simulink model "FSE"  (R2020a)
settings: Solver=ode45  StartTime=0.0  StopTime=2e3  RelTol=1e-3  EnableMultiTasking=on
PreLoadFcn:
  | FSE_PreLoadFcn
undefined symbols (not defined in the file): j
libraries: xbsIndex_r4 x138, dspmlti4 x2, xbsCopyrightNotice_r4 x1
(part 1 of 2)
settings Model: Creator=alexc  LastModifiedBy=viswanad
settings DataIOCC: LimitDataPoints=on  SaveFormat=Array  SignalLoggingSaveFormat=ModelDataLogs  ReturnWorkspaceOutputs=off  SignalLoggingName=sigsOut
settings OptimizationCC: BlockReduction=off  BooleanDataType=off  DefaultParameterBehavior=Inlined  ExpressionDepthLimit=2147483647  InitFltsAndDblsToZero=on  LifeSpan=inf
settings DebuggingCC: SaveWithParameterizedLinksMsg=none  UnderspecifiedInitializationDetection=Classic  MergeDetectMultiDrivingBlocksExec=none  SignalResolutionControl=TryResolveAllWithWarning  MultiTaskDSMMsg=warning  MultiTaskCondExecSysMsg=none  FcnCallInpInsideContextMsg=warning  AllowSymbolicDim=off  StateNameClashWarn=warning  SFUnexpectedBacktrackingDiag=warning  SFNoUnconditionalDefaultTransitionDiag=warning  SFExecutionAtInitializationDiag=none  ArithmeticOperatorsInVariantConditions=warning
settings HardwareCC: ProdBitPerPointer=32  ProdBitPerSizeT=32  ProdBitPerPtrDiffT=32  ProdLargestAtomicFloat=None  ProdIntDivRoundTo=Undefined  ProdEndianess=Unspecified  ProdWordSize=32  ProdHWDeviceType=32-bit Generic  TargetUnknown=on
settings ModelReferenceCC: PropagateSignalLabelsOutOfModel=off
settings SFSimCC: SimUseLocalCustomCode=off  CustomCodeUndefinedFunction=UseInterfaceOnly
settings RTWCC: Description=Generic Real-Time Target  RTWUseLocalCustomCode=off
settings CodeAppCC: StateflowObjectComments=on
settings GRTTargetCC: TargetFcnLib=ansi_tfl_tmw.mat  TargetLangStandard=C89/C90 (ANSI)  CombineOutputUpdateFcns=off  GRTInterface=on
settings ConfigComp: CovMetricSettings=dw  CovHtmlReporting=on  CovSaveCumulativeToWorkspaceVar=on  CovSaveSingleToWorkspaceVar=on  CovExternalEMLEnable=off

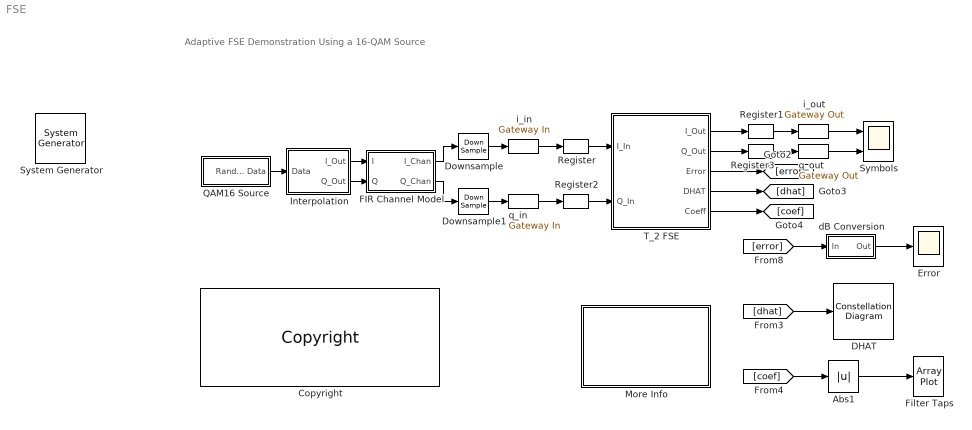
== system FSE ==
  note: Adaptive FSE Demonstration Using a 16-QAM Source
  " System Generator" : xbsIndex_r4/ System Generator  Tag=genX  xilinxfamily=kintex7  part=xc7k325t  speed=-3  package=fbg676  synthesis_tool=Vivado  clock_wrapper=Clock Enables  directory=./netlist  proj_type=Vivado  Synth_file=Vivado Synthesis Defaults  Impl_file=Vivado Implementation Defaults  testbench=off  simulink_period=1  sysclk_period=15  dcm_input_clock_period=10  incr_netlist=off  trim_vbits=Everywhere in SubSystem  dbl_ovrd=According to Block Masks  core_generation=According to Block Masks  run_coregen=off  deprecated_control=off  eval_field=0  block_type=sysgen
  Abs1 : Abs  SaturateOnIntegerOverflow=on
  Copyright : xbsCopyrightNotice_r4/Copyright  copyrighttext="Copyright (c) 2021  by  Xilinx, Inc. All rights reserved.<br><br>This file contains proprietary, confidential information of Xilinx, Inc., is distributed under license from Xilinx, Inc., and may be used, copied and/or disclosed only pursuant to the terms of a valid license agreement with Xilinx, Inc. Xilinx hereby grants you a license to use this file solely for design, simulation, implementation and creation of design files limited to Xilinx devices or technologies. Use with non-Xilinx devices or technologies is expressly prohibited and immediately terminates your license unless covered by a separate agreement.<br><br>Xilinx is providing this design, code, or information \"as-is\" solely for use in developing programs and solutions for Xilinx devices, with no obligation on the part of Xilinx to provide support. By providing this design, code, or information as one possible implementation of this feature, application or standard, Xilinx is making no representation that this implementation is free from any claims of infringement. You are responsible for obtaining any rights you may require for your implementation. Xilinx expressly disclaims any warranty whatsoever with respect to the adequacy of the implementation, including but not limited to any warranties or representations that this implementation is free from claims of infringement, implied warranties of merchantability or fitness for a particular purpose.<br><br>Xilinx products are not intended for use in life support appliances, devices, or systems. Use in such applications is expressly prohibited.<br><br>Any modifications that are made to the Source Code are done at the user's sole risk and will be unsupported.<br><br>This copyright and support notice must be retained as part of this text at all times. (c) Copyright 1995-2021 Xilinx, Inc. All rights reserved."  block_type=copyright
  DHAT : ConstellationDiagram
  Downsample : DownSample  RateOptions=Allow multirate processing
  Downsample1 : DownSample  RateOptions=Allow multirate processing
  Error : Scope
  FIR Channel Model : Subsystem  mask{chan=[1+j*0.1 .2 j*0.2 0 0 0 0 0 0 0]}
      mask prompts: chan "Channel"
  Filter Taps : ArrayPlot
  Interpolation : Subsystem
  More Info : Subsystem
      mask Display: disp('Double click\n for\n more information.')
  QAM16 Source : Subsystem
  Register{,1..3} (4 alike) : xbsIndex_r4/Register  init=0  rst=off  en=off  XmcBlockStatus=1  maskContainerNames=tabcontainer1  block_type=register  block_config=sysgen:Register_config
  Symbols : Scope  NumInputPorts=2
  T_2 FSE : Subsystem  mask{mu=.005}
  dB Conversion : Subsystem
  i_in : xbsIndex_r4/Gateway In  gui_display_data_type=Fixed-point  arith_type=Signed (2's comp)  n_bits=12  bin_pt=10  preci_type=Single  exp_width=8  frac_width=24  rows=1  columns=1  quantization="Round  (unbiased: +/- Inf)"  overflow=Saturate  period=2  UseAsADC=off  ADCChannel='1'  interface=None  automatic_assignment=on  address_offset=hex2dec('00')  intf_name=''  intf_description=''  default_value=0  timing_constraint=None  locs_specified=off  LOCs={}  io_standard={}  inherit_from_input=off  hdl_port=on  XmcBlockStatus=1  maskContainerNames=group4  block_type=gatewayin  block_config=sysgen:gateway_in_config
  i_out : xbsIndex_r4/Gateway Out  inherit_from_input=off  hdl_port=on  rows=1  columns=1  UseAsDAC=off  DACChannel='1'  interface=None  automatic_assignment=on  address_offset=hex2dec('00')  intf_name=''  intf_description=''  timing_constraint="Data Rate;  Set 'FAST' Attribute"  locs_specified=off  LOCs={}  io_standard={}  XmcBlockStatus=1  maskContainerNames=group4  block_type=gatewayout  block_config=sysgen:gateway_out_config
  q_in : xbsIndex_r4/Gateway In  gui_display_data_type=Fixed-point  arith_type=Signed (2's comp)  n_bits=12  bin_pt=10  preci_type=Single  exp_width=8  frac_width=24  rows=1  columns=1  quantization="Round  (unbiased: +/- Inf)"  overflow=Saturate  period=2  UseAsADC=off  ADCChannel='1'  interface=None  automatic_assignment=on  address_offset=hex2dec('00')  intf_name=''  intf_description=''  default_value=0  timing_constraint=None  locs_specified=off  LOCs={}  io_standard={}  inherit_from_input=off  hdl_port=on  XmcBlockStatus=1  maskContainerNames=group4  block_type=gatewayin  block_config=sysgen:gateway_in_config
  q_out : xbsIndex_r4/Gateway Out  inherit_from_input=off  hdl_port=on  rows=1  columns=1  UseAsDAC=off  DACChannel='1'  interface=None  automatic_assignment=on  address_offset=hex2dec('00')  intf_name=''  intf_description=''  timing_constraint="Data Rate;  Set 'FAST' Attribute"  locs_specified=off  LOCs={}  io_standard={}  XmcBlockStatus=1  maskContainerNames=group4  block_type=gatewayout  block_config=sysgen:gateway_out_config
  wires:
  QAM16 Source/1(" Random Data") -> Interpolation/1(Data)
  Interpolation/2(Q_Out) -> FIR Channel Model/2(Q)
  T_2 FSE/3(Error) -> [error]
  Downsample1/1 -> q_in/1
  Downsample/1 -> i_in/1
  Interpolation/1(I_Out) -> FIR Channel Model/1(I)
  T_2 FSE/2(Q_Out) -> Register3/1
  T_2 FSE/1(I_Out) -> Register1/1
  FIR Channel Model/1(I_Chan) -> Downsample/1
  FIR Channel Model/2(Q_Chan) -> Downsample1/1
  T_2 FSE/5(Coeff) -> [coef]
  i_in/1 -> Register/1
  Abs1/1 -> Filter Taps/1
  T_2 FSE/4(DHAT) -> [dhat]
  dB Conversion/1(Out) -> Error/1
  Register2/1 -> T_2 FSE/2(Q_In)
  Register1/1 -> i_out/1
  Register3/1 -> q_out/1
  q_in/1 -> Register2/1
  Register/1 -> T_2 FSE/1(I_In)
  [coef] -> Abs1/1
  [dhat] -> DHAT/1
  [error] -> dB Conversion/1(In)
  i_out/1 -> Symbols/1
  q_out/1 -> Symbols/2

== system FSE/FIR Channel Model ==
  I : Inport
  Q : Inport  Port=2
  Channel : Subsystem
  Channel1 : Subsystem
  Complex to Real-Imag1 : ComplexToRealImag
  Gain : Gain  Gain=j  SaturateOnIntegerOverflow=on  OutDataTypeStr=Inherit: Same as input  ParamDataTypeStr=Inherit: Same as input
  Random Number : RandomNumber  Variance=.01  SampleTime=100000
  Sum : Sum  Inputs=+++  InputSameDT=on  SaturateOnIntegerOverflow=on  OutDataTypeStr=Inherit: Same as first input
  I_Chan : Outport  VectorParamsAs1DForOutWhenUnconnected=off
  Q_Chan : Outport  Port=2  VectorParamsAs1DForOutWhenUnconnected=off
  wires:
  Channel1/1(yn) -> Gain/1
  Channel/1(yn) -> Sum/1
  Q/1 -> Channel1/1(xn)
  I/1 -> Channel/1(xn)
  Random Number/1 -> Sum/2
  Gain/1 -> Sum/3
  Sum/1 -> Complex to Real-Imag1/1
  Complex to Real-Imag1/2 -> Q_Chan/1
  Complex to Real-Imag1/1 -> I_Chan/1

== system FSE/Interpolation ==
  Data : Inport
  Complex to Real-Imag5 : ComplexToRealImag
  FIR Interpolation : dspmlti4/FIR Interpolation  FilterSource=Dialog parameters  PrivateCoeffs=0  h=sinc(-3:.25:3);  L=4  FilterObject=Hm_firinterp  framing=Allow multirate processing  outputBufInitCond=0  roundingMode=Floor  overflowMode=off  firstCoeffDataTypeStr=Inherit: Same word length as input  firstCoeffMin=[]  firstCoeffMax=[]  firstCoeffLastDataTypeStr=Inherit: Same word length as input  outputDataTypeStr=Inherit: Same as accumulator  outputMin=[]  outputMax=[]  outputLastDataTypeStr=Inherit: Same as accumulator
  FIR Interpolation1 : dspmlti4/FIR Interpolation  FilterSource=Dialog parameters  PrivateCoeffs=0  h=sinc(-3:.25:3);  L=4  FilterObject=Hm_firinterp  framing=Allow multirate processing  outputBufInitCond=0  roundingMode=Floor  overflowMode=off  firstCoeffDataTypeStr=Inherit: Same word length as input  firstCoeffMin=[]  firstCoeffMax=[]  firstCoeffLastDataTypeStr=Inherit: Same word length as input  outputDataTypeStr=Inherit: Same as accumulator  outputMin=[]  outputMax=[]  outputLastDataTypeStr=Inherit: Same as accumulator
  I_Out : Outport  VectorParamsAs1DForOutWhenUnconnected=off
  Q_Out : Outport  Port=2  VectorParamsAs1DForOutWhenUnconnected=off
  wires:
  Complex to Real-Imag5/2 -> FIR Interpolation1/1
  Complex to Real-Imag5/1 -> FIR Interpolation/1
  FIR Interpolation/1 -> I_Out/1
  Data/1 -> Complex to Real-Imag5/1
  FIR Interpolation1/1 -> Q_Out/1

== system FSE/More Info ==
  note: This design shows a T/2 adaptive Fractionally Space Equalizer (FSE)
      | operating on a 16-QAM data source with noise and filtering introduced
      | in the channel model.  The two 4-tap FIR filters are based on an
      | SRL16E-based MAC implementation.
      |
      | The DHAT scope provides an X-Y plot of the I and Q filter outputs from
      | within the FSE.  As the simulation progresses, these symbols will
      | converge as the error is reduced.  The magnitude of the filter coefficients
      | is shown in a vector scope as well.  Increasing the simulation duration
      | will allow better visualization of the adaptive FSE effects on the filter output.
      |
      |
      | For additional information on FSE:
      |
      | J.R. Treichler, I. Fijalkow, and C.R. Johnson, Jr.  "Fractionally Spaced
      | Equalizers"  IEEE Signal Processing Magazine, May 1996, pp. 65-81.
      |
      | Chris H. Dick, "Design and implementation of high-performance FPGA
      | signal processing datapaths for software-defined radios" VMEbus
      | Systems, August 2001.
  note: Adaptive FSE Demonstration Using a 16-QAM Source

== system FSE/QAM16 Source ==
  QAM16 - I : Subsystem
  QAM16 -Q : Subsystem
  Real-Imag to Complex : RealImagToComplex
  " Random Data" : Outport  VectorParamsAs1DForOutWhenUnconnected=off
  wires:
  QAM16 - I/1(I) -> Real-Imag to Complex/1
  QAM16 -Q/1(Q) -> Real-Imag to Complex/2
  Real-Imag to Complex/1 -> " Random Data"/1

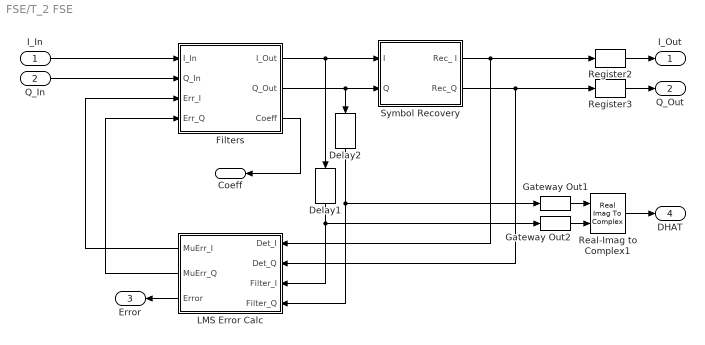
== system FSE/T_2 FSE ==
  I_In : Inport
  Q_In : Inport  Port=2
  Delay1 : xbsIndex_r4/Delay  rst=off  en=off  latency=2  reg_retiming=off  XmcBlockStatus=1  maskContainerNames=group1  block_type=delay  block_config=sysgen:Delay_config
  Delay2 : xbsIndex_r4/Delay  rst=off  en=off  latency=2  reg_retiming=off  XmcBlockStatus=1  maskContainerNames=group1  block_type=delay  block_config=sysgen:Delay_config
  Filters : Subsystem
  Gateway Out1 : xbsIndex_r4/Gateway Out  inherit_from_input=off  hdl_port=off  rows=1  columns=1  UseAsDAC=off  DACChannel='1'  interface=None  automatic_assignment=on  address_offset=hex2dec('00')  intf_name=''  intf_description=''  timing_constraint=None  locs_specified=off  LOCs={}  io_standard={}  XmcBlockStatus=1  maskContainerNames=group4  block_type=gatewayout  block_config=sysgen:gateway_out_config
  Gateway Out2 : xbsIndex_r4/Gateway Out  inherit_from_input=off  hdl_port=off  rows=1  columns=1  UseAsDAC=off  DACChannel='1'  interface=None  automatic_assignment=on  address_offset=hex2dec('00')  intf_name=''  intf_description=''  timing_constraint=None  locs_specified=off  LOCs={}  io_standard={}  XmcBlockStatus=1  maskContainerNames=group4  block_type=gatewayout  block_config=sysgen:gateway_out_config
  LMS Error Calc : Subsystem
  Real-Imag to Complex1 : RealImagToComplex
  Register2 : xbsIndex_r4/Register  init=0  rst=off  en=off  XmcBlockStatus=1  maskContainerNames=tabcontainer1  block_type=register  block_config=sysgen:Register_config
  Register3 : xbsIndex_r4/Register  init=0  rst=off  en=off  XmcBlockStatus=1  maskContainerNames=tabcontainer1  block_type=register  block_config=sysgen:Register_config
  Symbol Recovery : Subsystem
  I_Out : Outport  VectorParamsAs1DForOutWhenUnconnected=off
  Q_Out : Outport  Port=2  VectorParamsAs1DForOutWhenUnconnected=off
  Error : Outport  Port=3  VectorParamsAs1DForOutWhenUnconnected=off
  DHAT : Outport  Port=4  VectorParamsAs1DForOutWhenUnconnected=off
  Coeff : Outport  Port=5  VectorParamsAs1DForOutWhenUnconnected=off
  wires:
  Q_In/1 -> Filters/2(Q_In)
  LMS Error Calc/2(MuErr_Q) -> Filters/4(Err_Q)
  LMS Error Calc/1(MuErr_I) -> Filters/3(Err_I)
  Filters/1(I_Out) -> Delay1/1, Symbol Recovery/1(I)
  Symbol Recovery/2(Rec_Q) -> LMS Error Calc/2(Det_Q), Register3/1
  Symbol Recovery/1(Rec_ I) -> LMS Error Calc/1(Det_I), Register2/1
  Filters/2(Q_Out) -> Symbol Recovery/2(Q), Delay2/1
  I_In/1 -> Filters/1(I_In)
  Delay1/1 -> Gateway Out2/1, LMS Error Calc/3(Filter_I)
  Delay2/1 -> Gateway Out1/1, LMS Error Calc/4(Filter_Q)
  Real-Imag to Complex1/1 -> DHAT/1
  Gateway Out1/1 -> Real-Imag to Complex1/1
  Gateway Out2/1 -> Real-Imag to Complex1/2
  Filters/3(Coeff) -> Coeff/1
  LMS Error Calc/3(Error) -> Error/1
  Register2/1 -> I_Out/1
  Register3/1 -> Q_Out/1

== system FSE/dB Conversion ==
  In : Inport
  Abs : Abs  SaturateOnIntegerOverflow=on
  Constant : Constant  Value=0
  Constant1 : Constant
  Constant2 : Constant
  Gain1 : Gain  Gain=20  SaturateOnIntegerOverflow=on  OutDataTypeStr=Inherit: Same as input  ParamDataTypeStr=Inherit: Same as input
  Multiport Switch : MultiPortSwitch  Inputs=2  SaturateOnIntegerOverflow=on  InputSameDT=on
  Relational Operator : RelationalOperator  Operator===  RndMeth=Nearest  InputSameDT=on
  Sum : Sum  Inputs=|++  InputSameDT=on  SaturateOnIntegerOverflow=on  OutDataTypeStr=Inherit: Same as first input
  log10 : Math  Operator=log10  SignedPower=on  SaturateOnIntegerOverflow=on
  Out : Outport  VectorParamsAs1DForOutWhenUnconnected=off
  wires:
  Multiport Switch/1 -> log10/1
  Constant1/1 -> Multiport Switch/3
  Constant/1 -> Relational Operator/1
  Abs/1 -> Multiport Switch/2, Relational Operator/2
  Constant2/1 -> Sum/2
  Sum/1 -> Multiport Switch/1
  Relational Operator/1 -> Sum/1
  Gain1/1 -> Out/1
  In/1 -> Abs/1
  log10/1 -> Gain1/1

== system FSE/FIR Channel Model/Channel ==
  xn : Inport
  Chan Re : Subsystem
  yn : Outport  VectorParamsAs1DForOutWhenUnconnected=off
  wires:
  xn/1 -> Chan Re/1(Input)
  Chan Re/1(Output) -> yn/1

== system FSE/FIR Channel Model/Channel1 ==
  xn : Inport
  Chan Re : Subsystem
  yn : Outport  VectorParamsAs1DForOutWhenUnconnected=off
  wires:
  xn/1 -> Chan Re/1(Input)
  Chan Re/1(Output) -> yn/1

== system FSE/QAM16 Source/QAM16 - I ==
  Constant : Constant  Value=3
  Gain : Gain  Gain=2  SaturateOnIntegerOverflow=on  OutDataTypeStr=Inherit: Same as input  ParamDataTypeStr=Inherit: Same as input
  Gain1 : Gain  Gain=1/3  SaturateOnIntegerOverflow=on  OutDataTypeStr=Inherit: Same as input  ParamDataTypeStr=Inherit: Same as input
  Random Integer Generator : Subsystem  mask{M=4, seed=1, Ts=4}
      mask prompts: M "M-ary Number"; seed "Initial seed"; Ts "Sample Time"
  Sum : Sum  Inputs=|+-  InputSameDT=on  SaturateOnIntegerOverflow=on  OutDataTypeStr=Inherit: Same as first input
  I : Outport  VectorParamsAs1DForOutWhenUnconnected=off
  wires:
  Random Integer Generator/1(Out1) -> Gain/1
  Gain/1 -> Sum/1
  Constant/1 -> Sum/2
  Sum/1 -> Gain1/1
  Gain1/1 -> I/1

== system FSE/QAM16 Source/QAM16 -Q ==
  Constant : Constant  Value=3
  Gain : Gain  Gain=2  SaturateOnIntegerOverflow=on  OutDataTypeStr=Inherit: Same as input  ParamDataTypeStr=Inherit: Same as input
  Gain1 : Gain  Gain=1/3  SaturateOnIntegerOverflow=on  OutDataTypeStr=Inherit: Same as input  ParamDataTypeStr=Inherit: Same as input
  Random Integer Generator : Subsystem  mask{M=4, seed=4, Ts=4}
      mask prompts: M "M-ary Number"; seed "Initial seed"; Ts "Sample Time"
  Sum : Sum  Inputs=|+-  InputSameDT=on  SaturateOnIntegerOverflow=on  OutDataTypeStr=Inherit: Same as first input
  Q : Outport  VectorParamsAs1DForOutWhenUnconnected=off
  wires:
  Random Integer Generator/1(Out1) -> Gain/1
  Gain/1 -> Sum/1
  Constant/1 -> Sum/2
  Sum/1 -> Gain1/1
  Gain1/1 -> Q/1

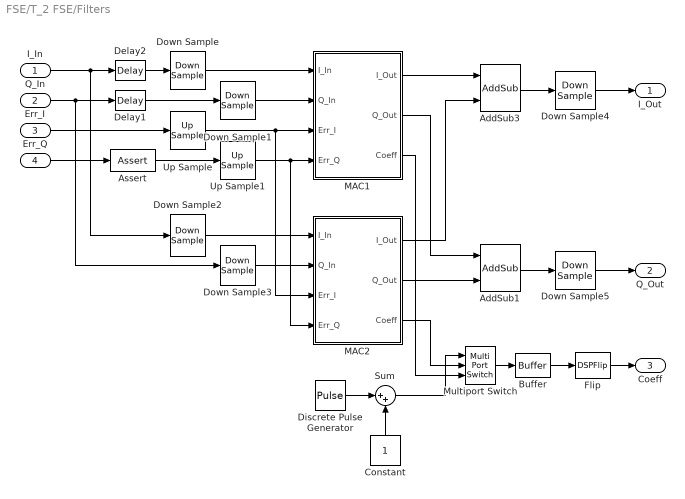
== system FSE/T_2 FSE/Filters ==
  I_In : Inport
  Q_In : Inport  Port=2
  Err_I : Inport  Port=3
  Err_Q : Inport  Port=4
  AddSub1 : xbsIndex_r4/AddSub  mode=Addition  use_carryin=off  use_carryout=off  en=off  latency=0  precision=User Defined  arith_type="Signed  (2's comp)"  n_bits=18  bin_pt=10  quantization="Round  (unbiased: +/- Inf)"  overflow=Saturate  use_behavioral_HDL=on  hw_selection=Fabric  pipelined=off  use_rpm=off  XmcBlockStatus=1  maskContainerNames=tabcontainer1  block_type=addsub  block_config=sysgen:Addsub_config
  AddSub3 : xbsIndex_r4/AddSub  mode=Addition  use_carryin=off  use_carryout=off  en=off  latency=0  precision=User Defined  arith_type="Signed  (2's comp)"  n_bits=18  bin_pt=10  quantization="Round  (unbiased: +/- Inf)"  overflow=Saturate  use_behavioral_HDL=on  hw_selection=Fabric  pipelined=off  use_rpm=off  XmcBlockStatus=1  maskContainerNames=tabcontainer1  block_type=addsub  block_config=sysgen:Addsub_config
  Assert : xbsIndex_r4/Assert  assert_type=off  type_source=Explicitly  gui_display_data_type=Fixed-point  arith_type=Unsigned  n_bits=8  bin_pt=2  preci_type=Single  exp_width=8  frac_width=24  assert_rate=on  rate_source=Explicitly  period=4  output_port=on  XmcBlockStatus=1  maskContainerNames=group1  block_type=assert  block_config=sysgen:assert_config
  Buffer : Buffer  N=8
  Constant : Constant
  Delay1 : xbsIndex_r4/Delay  rst=off  en=off  latency=1  reg_retiming=off  XmcBlockStatus=1  maskContainerNames=group1  block_type=delay  block_config=sysgen:Delay_config
  Delay2 : xbsIndex_r4/Delay  rst=off  en=off  latency=1  reg_retiming=off  XmcBlockStatus=1  maskContainerNames=group1  block_type=delay  block_config=sysgen:Delay_config
  Discrete Pulse Generator : DiscretePulseGenerator  SampleTime=.5
  Down Sample : xbsIndex_r4/Down Sample  sample_ratio=2  sample_phase="Last Value of Frame  (most efficient)"  en=off  rst=off  latency=1  XmcBlockStatus=1  maskContainerNames=group1  block_type=dsamp  block_config=sysgen:Downsample_config
  Down Sample1 : xbsIndex_r4/Down Sample  sample_ratio=2  sample_phase="Last Value of Frame  (most efficient)"  en=off  rst=off  latency=1  XmcBlockStatus=1  maskContainerNames=group1  block_type=dsamp  block_config=sysgen:Downsample_config
  Down Sample2 : xbsIndex_r4/Down Sample  sample_ratio=2  sample_phase="Last Value of Frame  (most efficient)"  en=off  rst=off  latency=2  XmcBlockStatus=1  maskContainerNames=group1  block_type=dsamp  block_config=sysgen:Downsample_config
  Down Sample3 : xbsIndex_r4/Down Sample  sample_ratio=2  sample_phase="Last Value of Frame  (most efficient)"  en=off  rst=off  latency=2  XmcBlockStatus=1  maskContainerNames=group1  block_type=dsamp  block_config=sysgen:Downsample_config
  Down Sample4 : xbsIndex_r4/Down Sample  sample_ratio=4  sample_phase="Last Value of Frame  (most efficient)"  en=off  rst=off  latency=1  XmcBlockStatus=1  maskContainerNames=group1  block_type=dsamp  block_config=sysgen:Downsample_config
  Down Sample5 : xbsIndex_r4/Down Sample  sample_ratio=4  sample_phase="Last Value of Frame  (most efficient)"  en=off  rst=off  latency=1  XmcBlockStatus=1  maskContainerNames=group1  block_type=dsamp  block_config=sysgen:Downsample_config
  Flip : DSPFlip
  MAC1 : Subsystem
  MAC2 : Subsystem
  Multiport Switch : MultiPortSwitch  Inputs=2  SaturateOnIntegerOverflow=on  InputSameDT=on
  Sum : Sum  Inputs=|++  InputSameDT=on  SaturateOnIntegerOverflow=on  OutDataTypeStr=Inherit: Same as first input
  Up Sample : xbsIndex_r4/Up Sample  sample_ratio=4  copy_samples=on  en=off  latency=0  XmcBlockStatus=1  maskContainerNames=group1  block_type=usamp  block_config=sysgen:Upsample_config
  Up Sample1 : xbsIndex_r4/Up Sample  sample_ratio=4  copy_samples=on  en=off  latency=0  XmcBlockStatus=1  maskContainerNames=group1  block_type=usamp  block_config=sysgen:Upsample_config
  I_Out : Outport  VectorParamsAs1DForOutWhenUnconnected=off
  Q_Out : Outport  Port=2  VectorParamsAs1DForOutWhenUnconnected=off
  Coeff : Outport  Port=3  VectorParamsAs1DForOutWhenUnconnected=off
  wires:
  Down Sample3/1 -> MAC2/2(Q_In)
  Down Sample1/1 -> MAC1/2(Q_In)
  Down Sample/1 -> MAC1/1(I_In)
  AddSub3/1 -> Down Sample4/1
  MAC1/2(Q_Out) -> AddSub1/1
  MAC2/1(I_Out) -> AddSub3/2
  MAC2/2(Q_Out) -> AddSub1/2
  AddSub1/1 -> Down Sample5/1
  Multiport Switch/1 -> Buffer/1
  Constant/1 -> Sum/2
  Discrete Pulse Generator/1 -> Sum/1
  Sum/1 -> Multiport Switch/1
  MAC1/3(Coeff) -> Multiport Switch/3
  MAC2/3(Coeff) -> Multiport Switch/2
  Buffer/1 -> Flip/1
  Flip/1 -> Coeff/1
  Down Sample4/1 -> I_Out/1
  Down Sample5/1 -> Q_Out/1
  Delay2/1 -> Down Sample/1
  Delay1/1 -> Down Sample1/1
  Down Sample2/1 -> MAC2/1(I_In)
  Err_Q/1 -> Assert/1
  Err_I/1 -> Up Sample/1
  Q_In/1 -> Delay1/1, Down Sample3/1
  I_In/1 -> Delay2/1, Down Sample2/1
  MAC1/1(I_Out) -> AddSub3/1
  Up Sample/1 -> MAC1/3(Err_I), MAC2/3(Err_I)
  Up Sample1/1 -> MAC1/4(Err_Q), MAC2/4(Err_Q)
  Assert/1 -> Up Sample1/1

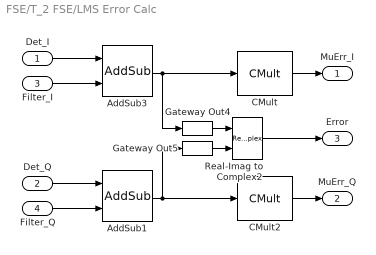
== system FSE/T_2 FSE/LMS Error Calc ==
  Det_I : Inport
  Det_Q : Inport  Port=2
  Filter_I : Inport  Port=3
  Filter_Q : Inport  Port=4
  AddSub1 : xbsIndex_r4/AddSub  mode=Subtraction  use_carryin=off  use_carryout=off  en=off  latency=1  precision=Full  arith_type="Signed  (2's comp)"  n_bits=36  bin_pt=28  quantization="Round  (unbiased: +/- Inf)"  overflow=Saturate  use_behavioral_HDL=on  hw_selection=Fabric  pipelined=off  use_rpm=off  XmcBlockStatus=1  maskContainerNames=tabcontainer1  block_type=addsub  block_config=sysgen:Addsub_config
  AddSub3 : xbsIndex_r4/AddSub  mode=Subtraction  use_carryin=off  use_carryout=off  en=off  latency=1  precision=Full  arith_type="Signed  (2's comp)"  n_bits=36  bin_pt=28  quantization="Round  (unbiased: +/- Inf)"  overflow=Saturate  use_behavioral_HDL=on  hw_selection=Fabric  pipelined=off  use_rpm=off  XmcBlockStatus=1  maskContainerNames=tabcontainer1  block_type=addsub  block_config=sysgen:Addsub_config
  CMult : xbsIndex_r4/CMult  const=mu  gui_display_data_type=Fixed-point  const_n_bits=18  const_bin_pt=16  float_type=Single  exp_bits=8  fraction_bits=24  en=off  latency=1  precision=User Defined  arith_type="Signed  (2's comp)"  n_bits=18  bin_pt=15  quantization="Round  (unbiased: +/- Inf)"  overflow=Wrap  use_behavioral_HDL=off  mem_type=Distributed RAM  pipeline=off  use_rpm=off  placement_style=Rectangular Shape  XmcBlockStatus=1  maskContainerNames=tabcontainer1  block_type=cmult  block_config=sysgen:CMult_config
      settings: infoedit=[]
  CMult2 : xbsIndex_r4/CMult  const=-mu  gui_display_data_type=Fixed-point  const_n_bits=18  const_bin_pt=16  float_type=Single  exp_bits=8  fraction_bits=24  en=off  latency=1  precision=User Defined  arith_type="Signed  (2's comp)"  n_bits=18  bin_pt=15  quantization="Round  (unbiased: +/- Inf)"  overflow=Wrap  use_behavioral_HDL=off  mem_type=Distributed RAM  pipeline=off  use_rpm=off  placement_style=Rectangular Shape  XmcBlockStatus=1  maskContainerNames=tabcontainer1  block_type=cmult  block_config=sysgen:CMult_config
      settings: infoedit=[]
  Gateway Out4 : xbsIndex_r4/Gateway Out  inherit_from_input=off  hdl_port=off  rows=1  columns=1  UseAsDAC=off  DACChannel='1'  interface=None  automatic_assignment=on  address_offset=hex2dec('00')  intf_name=''  intf_description=''  timing_constraint=None  locs_specified=off  LOCs={}  io_standard={}  XmcBlockStatus=1  maskContainerNames=group4  block_type=gatewayout  block_config=sysgen:gateway_out_config
  Gateway Out5 : xbsIndex_r4/Gateway Out  inherit_from_input=off  hdl_port=off  rows=1  columns=1  UseAsDAC=off  DACChannel='1'  interface=None  automatic_assignment=on  address_offset=hex2dec('00')  intf_name=''  intf_description=''  timing_constraint=None  locs_specified=off  LOCs={}  io_standard={}  XmcBlockStatus=1  maskContainerNames=group4  block_type=gatewayout  block_config=sysgen:gateway_out_config
  Real-Imag to Complex2 : RealImagToComplex
  MuErr_I : Outport  VectorParamsAs1DForOutWhenUnconnected=off
  MuErr_Q : Outport  Port=2  VectorParamsAs1DForOutWhenUnconnected=off
  Error : Outport  Port=3  VectorParamsAs1DForOutWhenUnconnected=off
  wires:
  CMult2/1 -> MuErr_Q/1
  CMult/1 -> MuErr_I/1
  AddSub3/1 -> CMult/1, Gateway Out4/1
  AddSub1/1 -> Gateway Out5/1, CMult2/1
  Det_Q/1 -> AddSub1/1
  Filter_Q/1 -> AddSub1/2
  Det_I/1 -> AddSub3/1
  Filter_I/1 -> AddSub3/2
  Gateway Out5/1 -> Real-Imag to Complex2/2
  Gateway Out4/1 -> Real-Imag to Complex2/1
  Real-Imag to Complex2/1 -> Error/1

== system FSE/T_2 FSE/Symbol Recovery ==
  I : Inport
  Q : Inport  Port=2
  I Map : Subsystem
  Q Map : Subsystem
  Rec_ I : Outport  VectorParamsAs1DForOutWhenUnconnected=off
  Rec_Q : Outport  Port=2  VectorParamsAs1DForOutWhenUnconnected=off
  wires:
  Q/1 -> Q Map/1(Q_In)
  I/1 -> I Map/1(I_In)
  I Map/1(Rec_I) -> Rec_ I/1
  Q Map/1(Rec_Q) -> Rec_Q/1

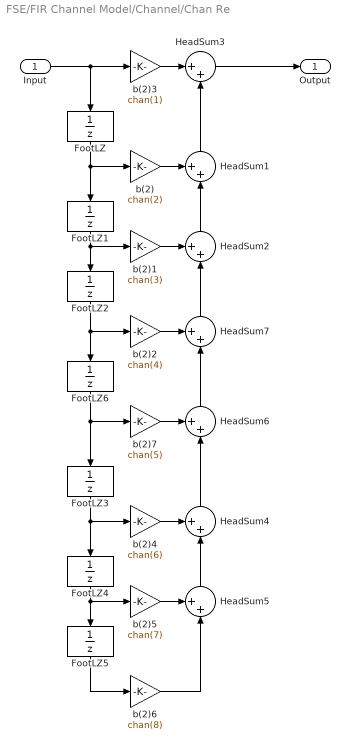
== system FSE/FIR Channel Model/Channel/Chan Re ==
  Input : Inport
  FootLZ : UnitDelay  HasFrameUpgradeWarning=on
  FootLZ{1..2,4..6} (5 alike) : UnitDelay  SampleTime=-1  HasFrameUpgradeWarning=on
  FootLZ3 : UnitDelay  HasFrameUpgradeWarning=on
  HeadSum{1..2,4..7} (6 alike) : Sum  Inputs=++|  InputSameDT=on  SaturateOnIntegerOverflow=on  OutDataTypeStr=Inherit: Same as first input
  HeadSum3 : Sum  Inputs=|++  InputSameDT=on  SaturateOnIntegerOverflow=on  OutDataTypeStr=Inherit: Same as first input
  b(2) : Gain  Gain=chan(2)  SaturateOnIntegerOverflow=on  OutDataTypeStr=Inherit: Same as input  ParamDataTypeStr=Inherit: Same as input
  b(2)1 : Gain  Gain=chan(3)  SaturateOnIntegerOverflow=on  OutDataTypeStr=Inherit: Same as input  ParamDataTypeStr=Inherit: Same as input
  b(2)2 : Gain  Gain=chan(4)  SaturateOnIntegerOverflow=on  OutDataTypeStr=Inherit: Same as input  ParamDataTypeStr=Inherit: Same as input
  b(2)3 : Gain  Gain=chan(1)  SaturateOnIntegerOverflow=on  OutDataTypeStr=Inherit: Same as input  ParamDataTypeStr=Inherit: Same as input
  b(2)4 : Gain  Gain=chan(6)  SaturateOnIntegerOverflow=on  OutDataTypeStr=Inherit: Same as input  ParamDataTypeStr=Inherit: Same as input
  b(2)5 : Gain  Gain=chan(7)  SaturateOnIntegerOverflow=on  OutDataTypeStr=Inherit: Same as input  ParamDataTypeStr=Inherit: Same as input
  b(2)6 : Gain  Gain=chan(8)  SaturateOnIntegerOverflow=on  OutDataTypeStr=Inherit: Same as input  ParamDataTypeStr=Inherit: Same as input
  b(2)7 : Gain  Gain=chan(5)  SaturateOnIntegerOverflow=on  OutDataTypeStr=Inherit: Same as input  ParamDataTypeStr=Inherit: Same as input
  Output : Outport  VectorParamsAs1DForOutWhenUnconnected=off
  wires:
  HeadSum6/1 -> HeadSum7/2
  HeadSum4/1 -> HeadSum6/2
  HeadSum7/1 -> HeadSum2/2
  b(2)2/1 -> HeadSum7/1
  FootLZ6/1 -> FootLZ3/1, b(2)7/1
  FootLZ3/1 -> b(2)4/1, FootLZ4/1
  FootLZ4/1 -> FootLZ5/1, b(2)5/1
  FootLZ5/1 -> b(2)6/1
  b(2)4/1 -> HeadSum4/1
  b(2)5/1 -> HeadSum5/1
  HeadSum5/1 -> HeadSum4/2
  b(2)6/1 -> HeadSum5/2
  b(2)7/1 -> HeadSum6/1
  FootLZ2/1 -> FootLZ6/1, b(2)2/1
  FootLZ/1 -> b(2)/1, FootLZ1/1
  FootLZ1/1 -> FootLZ2/1, b(2)1/1
  b(2)/1 -> HeadSum1/1
  b(2)1/1 -> HeadSum2/1
  HeadSum2/1 -> HeadSum1/2
  Input/1 -> FootLZ/1, b(2)3/1
  b(2)3/1 -> HeadSum3/1
  HeadSum1/1 -> HeadSum3/2
  HeadSum3/1 -> Output/1

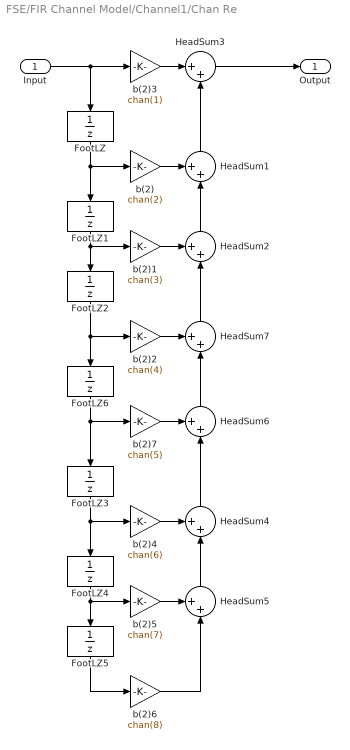
== system FSE/FIR Channel Model/Channel1/Chan Re ==
  Input : Inport
  FootLZ : UnitDelay  HasFrameUpgradeWarning=on
  FootLZ{1..2,4..6} (5 alike) : UnitDelay  SampleTime=-1  HasFrameUpgradeWarning=on
  FootLZ3 : UnitDelay  HasFrameUpgradeWarning=on
  HeadSum{1..2,4..7} (6 alike) : Sum  Inputs=++|  InputSameDT=on  SaturateOnIntegerOverflow=on  OutDataTypeStr=Inherit: Same as first input
  HeadSum3 : Sum  Inputs=|++  InputSameDT=on  SaturateOnIntegerOverflow=on  OutDataTypeStr=Inherit: Same as first input
  b(2) : Gain  Gain=chan(2)  SaturateOnIntegerOverflow=on  OutDataTypeStr=Inherit: Same as input  ParamDataTypeStr=Inherit: Same as input
  b(2)1 : Gain  Gain=chan(3)  SaturateOnIntegerOverflow=on  OutDataTypeStr=Inherit: Same as input  ParamDataTypeStr=Inherit: Same as input
  b(2)2 : Gain  Gain=chan(4)  SaturateOnIntegerOverflow=on  OutDataTypeStr=Inherit: Same as input  ParamDataTypeStr=Inherit: Same as input
  b(2)3 : Gain  Gain=chan(1)  SaturateOnIntegerOverflow=on  OutDataTypeStr=Inherit: Same as input  ParamDataTypeStr=Inherit: Same as input
  b(2)4 : Gain  Gain=chan(6)  SaturateOnIntegerOverflow=on  OutDataTypeStr=Inherit: Same as input  ParamDataTypeStr=Inherit: Same as input
  b(2)5 : Gain  Gain=chan(7)  SaturateOnIntegerOverflow=on  OutDataTypeStr=Inherit: Same as input  ParamDataTypeStr=Inherit: Same as input
  b(2)6 : Gain  Gain=chan(8)  SaturateOnIntegerOverflow=on  OutDataTypeStr=Inherit: Same as input  ParamDataTypeStr=Inherit: Same as input
  b(2)7 : Gain  Gain=chan(5)  SaturateOnIntegerOverflow=on  OutDataTypeStr=Inherit: Same as input  ParamDataTypeStr=Inherit: Same as input
  Output : Outport  VectorParamsAs1DForOutWhenUnconnected=off
  wires:
  b(2)2/1 -> HeadSum7/1
  HeadSum7/1 -> HeadSum2/2
  HeadSum6/1 -> HeadSum7/2
  FootLZ6/1 -> b(2)7/1, FootLZ3/1
  FootLZ2/1 -> FootLZ6/1, b(2)2/1
  FootLZ3/1 -> b(2)4/1, FootLZ4/1
  FootLZ4/1 -> FootLZ5/1, b(2)5/1
  FootLZ5/1 -> b(2)6/1
  b(2)4/1 -> HeadSum4/1
  b(2)5/1 -> HeadSum5/1
  HeadSum5/1 -> HeadSum4/2
  b(2)6/1 -> HeadSum5/2
  b(2)7/1 -> HeadSum6/1
  HeadSum4/1 -> HeadSum6/2
  FootLZ/1 -> b(2)/1, FootLZ1/1
  FootLZ1/1 -> FootLZ2/1, b(2)1/1
  b(2)/1 -> HeadSum1/1
  b(2)1/1 -> HeadSum2/1
  HeadSum2/1 -> HeadSum1/2
  Input/1 -> FootLZ/1, b(2)3/1
  b(2)3/1 -> HeadSum3/1
  HeadSum1/1 -> HeadSum3/2
  HeadSum3/1 -> Output/1

== system FSE/QAM16 Source/QAM16 - I/Random Integer Generator ==
  Rounding Function : Rounding  Operator=round
  Uniform Random Number : UniformRandomNumber  Minimum=-0.49  Maximum=M-1 + 0.49  Seed=seed  SampleTime=Ts
  Out1 : Outport  VectorParamsAs1DForOutWhenUnconnected=off
  wires:
  Rounding Function/1 -> Out1/1
  Uniform Random Number/1 -> Rounding Function/1

== system FSE/QAM16 Source/QAM16 -Q/Random Integer Generator ==
  Rounding Function : Rounding  Operator=round
  Uniform Random Number : UniformRandomNumber  Minimum=-0.49  Maximum=M-1 + 0.49  Seed=seed  SampleTime=Ts
  Out1 : Outport  VectorParamsAs1DForOutWhenUnconnected=off
  wires:
  Rounding Function/1 -> Out1/1
  Uniform Random Number/1 -> Rounding Function/1

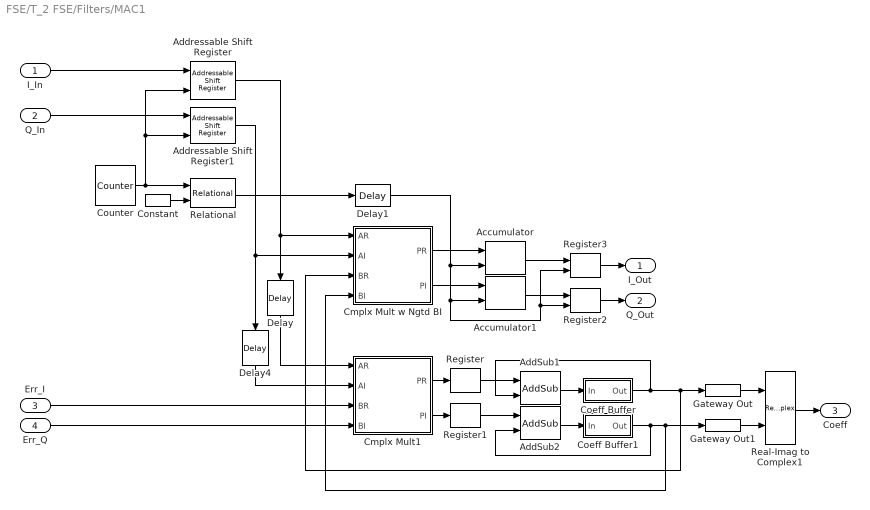
== system FSE/T_2 FSE/Filters/MAC1 ==
  I_In : Inport
  Q_In : Inport  Port=2
  Err_I : Inport  Port=3
  Err_Q : Inport  Port=4
  Accumulator : xbsIndex_r4/Accumulator  operation=Add  n_bits=36  overflow=Wrap  scale=1  rst=on  hasbypass=on  en=off  latency=1  msb_inp=100  msb=100  lsb=-100  use_behavioral_HDL=on  implementation=Fabric  XmcBlockStatus=1  maskContainerNames=group3  block_type=accum  block_config=sysgen:Accum_config
  Accumulator1 : xbsIndex_r4/Accumulator  operation=Add  n_bits=36  overflow=Wrap  scale=1  rst=on  hasbypass=on  en=off  latency=1  msb_inp=100  msb=100  lsb=-100  use_behavioral_HDL=on  implementation=Fabric  XmcBlockStatus=1  maskContainerNames=group3  block_type=accum  block_config=sysgen:Accum_config
  AddSub1 : xbsIndex_r4/AddSub  mode=Addition  use_carryin=off  use_carryout=off  en=off  latency=0  precision=User Defined  arith_type="Signed  (2's comp)"  n_bits=18  bin_pt=10  quantization="Round  (unbiased: +/- Inf)"  overflow=Saturate  use_behavioral_HDL=on  hw_selection=Fabric  pipelined=off  use_rpm=off  XmcBlockStatus=1  maskContainerNames=tabcontainer1  block_type=addsub  block_config=sysgen:Addsub_config
  AddSub2 : xbsIndex_r4/AddSub  mode=Addition  use_carryin=off  use_carryout=off  en=off  latency=0  precision=User Defined  arith_type="Signed  (2's comp)"  n_bits=18  bin_pt=10  quantization="Round  (unbiased: +/- Inf)"  overflow=Saturate  use_behavioral_HDL=on  hw_selection=Fabric  pipelined=off  use_rpm=off  XmcBlockStatus=1  maskContainerNames=tabcontainer1  block_type=addsub  block_config=sysgen:Addsub_config
  Addressable Shift Register : xbsIndex_r4/Addressable Shift Register  infer_latency=on  depth=2  initVector=0  en=off  use_behavioral_HDL=off  Optimization=Resource  use_rpm=off  XmcBlockStatus=1  maskContainerNames=group1  block_type=addrsr  block_config=sysgen:Addrsr_config
  Addressable Shift Register1 : xbsIndex_r4/Addressable Shift Register  infer_latency=on  depth=2  initVector=0  en=off  use_behavioral_HDL=off  Optimization=Resource  use_rpm=off  XmcBlockStatus=1  maskContainerNames=group1  block_type=addrsr  block_config=sysgen:Addrsr_config
  Cmplx Mult w Ngtd BI : Subsystem
  Cmplx Mult1 : Subsystem
  Coeff Buffer : Subsystem
  Coeff Buffer1 : Subsystem
  Constant : xbsIndex_r4/Constant  const=0  gui_display_data_type=Fixed-point  arith_type=Unsigned  n_bits=1  bin_pt=0  preci_type=Single  exp_width=8  frac_width=24  explicit_period=off  period=1  XmcBlockStatus=1  maskContainerNames=tabcontainer1  block_type=constant  block_config=sysgen:Constant_config
  Counter : xbsIndex_r4/Counter  cnt_type=Free Running  cnt_to=4  operation=Up  start_count=3  cnt_by_val=1  arith_type=Unsigned  n_bits=2  bin_pt=0  load_pin=off  rst=off  en=off  explicit_period=on  period=1  use_behavioral_HDL=off  implementation=Fabric  use_rpm=off  XmcBlockStatus=1  maskContainerNames=group1  block_type=counter  block_config=sysgen:Counter_config
  Delay : xbsIndex_r4/Delay  rst=off  en=off  latency=27  reg_retiming=off  XmcBlockStatus=1  maskContainerNames=group1  block_type=delay  block_config=sysgen:Delay_config
  Delay1 : xbsIndex_r4/Delay  rst=off  en=off  latency=3  reg_retiming=off  XmcBlockStatus=1  maskContainerNames=group1  block_type=delay  block_config=sysgen:Delay_config
  Delay4 : xbsIndex_r4/Delay  rst=off  en=off  latency=27  reg_retiming=off  XmcBlockStatus=1  maskContainerNames=group1  block_type=delay  block_config=sysgen:Delay_config
  Gateway Out : xbsIndex_r4/Gateway Out  inherit_from_input=off  hdl_port=off  rows=1  columns=1  UseAsDAC=off  DACChannel='1'  interface=None  automatic_assignment=on  address_offset=hex2dec('00')  intf_name=''  intf_description=''  timing_constraint=None  locs_specified=off  LOCs={}  io_standard={}  XmcBlockStatus=1  maskContainerNames=group4  block_type=gatewayout  block_config=sysgen:gateway_out_config
  Gateway Out1 : xbsIndex_r4/Gateway Out  inherit_from_input=off  hdl_port=off  rows=1  columns=1  UseAsDAC=off  DACChannel='1'  interface=None  automatic_assignment=on  address_offset=hex2dec('00')  intf_name=''  intf_description=''  timing_constraint=None  locs_specified=off  LOCs={}  io_standard={}  XmcBlockStatus=1  maskContainerNames=group4  block_type=gatewayout  block_config=sysgen:gateway_out_config
  Real-Imag to Complex1 : RealImagToComplex
  Register : xbsIndex_r4/Register  init=0  rst=off  en=off  XmcBlockStatus=1  maskContainerNames=tabcontainer1  block_type=register  block_config=sysgen:Register_config
  Register1 : xbsIndex_r4/Register  init=0  rst=off  en=off  XmcBlockStatus=1  maskContainerNames=tabcontainer1  block_type=register  block_config=sysgen:Register_config
  Register2 : xbsIndex_r4/Register  init=0  rst=off  en=on  XmcBlockStatus=1  maskContainerNames=tabcontainer1  block_type=register  block_config=sysgen:Register_config
  Register3 : xbsIndex_r4/Register  init=0  rst=off  en=on  XmcBlockStatus=1  maskContainerNames=tabcontainer1  block_type=register  block_config=sysgen:Register_config
  Relational : xbsIndex_r4/Relational  mode=a=b  op_type=Bool  en=off  latency=0  XmcBlockStatus=1  maskContainerNames=tabcontainer1  block_type=relational  block_config=sysgen:Relational_config
  I_Out : Outport  VectorParamsAs1DForOutWhenUnconnected=off
  Q_Out : Outport  Port=2  VectorParamsAs1DForOutWhenUnconnected=off
  Coeff : Outport  Port=3  VectorParamsAs1DForOutWhenUnconnected=off
  wires:
  Delay4/1 -> Cmplx Mult1/2(AI)
  Delay/1 -> Cmplx Mult1/1(AR)
  Accumulator/1 -> Register3/1
  Delay1/1 -> Accumulator/2, Accumulator1/2, Register3/2, Register2/2
  Cmplx Mult w Ngtd BI/1(PR) -> Accumulator/1
  Cmplx Mult w Ngtd BI/2(PI) -> Accumulator1/1
  Accumulator1/1 -> Register2/1
  Coeff Buffer1/1(Out) -> Gateway Out1/1, Cmplx Mult w Ngtd BI/4(BI), AddSub2/2
  Coeff Buffer/1(Out) -> AddSub1/2, Gateway Out/1, Cmplx Mult w Ngtd BI/3(BR)
  Counter/1 -> Addressable Shift Register1/2, Addressable Shift Register/2, Relational/1
  AddSub2/1 -> Coeff Buffer1/1(In)
  AddSub1/1 -> Coeff Buffer/1(In)
  Gateway Out/1 -> Real-Imag to Complex1/1
  Gateway Out1/1 -> Real-Imag to Complex1/2
  Real-Imag to Complex1/1 -> Coeff/1
  Err_I/1 -> Cmplx Mult1/3(BR)
  Err_Q/1 -> Cmplx Mult1/4(BI)
  Cmplx Mult1/2(PI) -> Register1/1
  Cmplx Mult1/1(PR) -> Register/1
  Addressable Shift Register/1 -> Delay/1, Cmplx Mult w Ngtd BI/1(AR)
  I_In/1 -> Addressable Shift Register/1
  Q_In/1 -> Addressable Shift Register1/1
  Addressable Shift Register1/1 -> Delay4/1, Cmplx Mult w Ngtd BI/2(AI)
  Register1/1 -> AddSub2/1
  Register/1 -> AddSub1/1
  Register3/1 -> I_Out/1
  Register2/1 -> Q_Out/1
  Relational/1 -> Delay1/1
  Constant/1 -> Relational/2

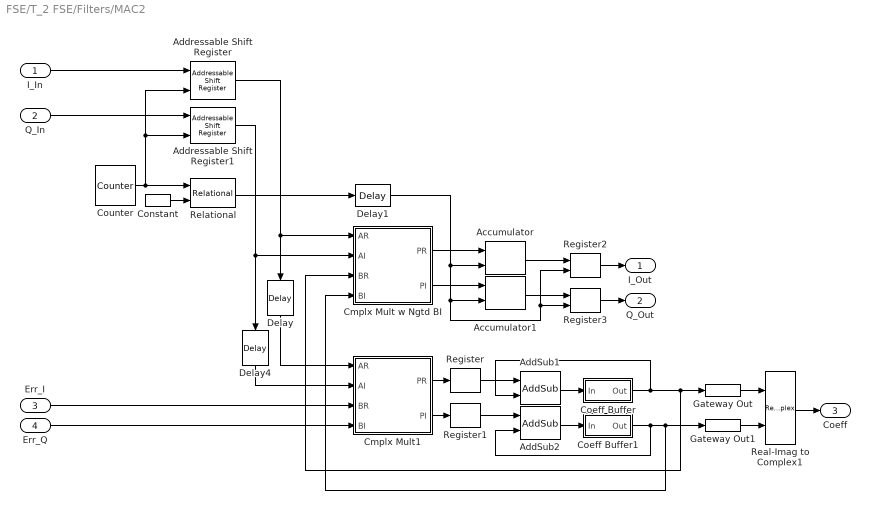
== system FSE/T_2 FSE/Filters/MAC2 ==
  I_In : Inport
  Q_In : Inport  Port=2
  Err_I : Inport  Port=3
  Err_Q : Inport  Port=4
  Accumulator : xbsIndex_r4/Accumulator  operation=Add  n_bits=36  overflow=Wrap  scale=1  rst=on  hasbypass=on  en=off  latency=1  msb_inp=100  msb=100  lsb=-100  use_behavioral_HDL=on  implementation=Fabric  XmcBlockStatus=1  maskContainerNames=group3  block_type=accum  block_config=sysgen:Accum_config
  Accumulator1 : xbsIndex_r4/Accumulator  operation=Add  n_bits=36  overflow=Wrap  scale=1  rst=on  hasbypass=on  en=off  latency=1  msb_inp=100  msb=100  lsb=-100  use_behavioral_HDL=on  implementation=Fabric  XmcBlockStatus=1  maskContainerNames=group3  block_type=accum  block_config=sysgen:Accum_config
  AddSub1 : xbsIndex_r4/AddSub  mode=Addition  use_carryin=off  use_carryout=off  en=off  latency=0  precision=User Defined  arith_type="Signed  (2's comp)"  n_bits=18  bin_pt=10  quantization="Round  (unbiased: +/- Inf)"  overflow=Saturate  use_behavioral_HDL=on  hw_selection=Fabric  pipelined=off  use_rpm=off  XmcBlockStatus=1  maskContainerNames=tabcontainer1  block_type=addsub  block_config=sysgen:Addsub_config
  AddSub2 : xbsIndex_r4/AddSub  mode=Addition  use_carryin=off  use_carryout=off  en=off  latency=0  precision=User Defined  arith_type="Signed  (2's comp)"  n_bits=18  bin_pt=10  quantization="Round  (unbiased: +/- Inf)"  overflow=Saturate  use_behavioral_HDL=on  hw_selection=Fabric  pipelined=off  use_rpm=off  XmcBlockStatus=1  maskContainerNames=tabcontainer1  block_type=addsub  block_config=sysgen:Addsub_config
  Addressable Shift Register : xbsIndex_r4/Addressable Shift Register  infer_latency=on  depth=2  initVector=0  en=off  use_behavioral_HDL=off  Optimization=Resource  use_rpm=off  XmcBlockStatus=1  maskContainerNames=group1  block_type=addrsr  block_config=sysgen:Addrsr_config
  Addressable Shift Register1 : xbsIndex_r4/Addressable Shift Register  infer_latency=on  depth=2  initVector=0  en=off  use_behavioral_HDL=off  Optimization=Resource  use_rpm=off  XmcBlockStatus=1  maskContainerNames=group1  block_type=addrsr  block_config=sysgen:Addrsr_config
  Cmplx Mult w Ngtd BI : Subsystem
  Cmplx Mult1 : Subsystem
  Coeff Buffer : Subsystem
  Coeff Buffer1 : Subsystem
  Constant : xbsIndex_r4/Constant  const=0  gui_display_data_type=Fixed-point  arith_type=Unsigned  n_bits=1  bin_pt=0  preci_type=Single  exp_width=8  frac_width=24  explicit_period=off  period=1  XmcBlockStatus=1  maskContainerNames=tabcontainer1  block_type=constant  block_config=sysgen:Constant_config
  Counter : xbsIndex_r4/Counter  cnt_type=Free Running  cnt_to=4  operation=Up  start_count=3  cnt_by_val=1  arith_type=Unsigned  n_bits=2  bin_pt=0  load_pin=off  rst=off  en=off  explicit_period=on  period=1  use_behavioral_HDL=off  implementation=Fabric  use_rpm=off  XmcBlockStatus=1  maskContainerNames=group1  block_type=counter  block_config=sysgen:Counter_config
  Delay : xbsIndex_r4/Delay  rst=off  en=off  latency=27  reg_retiming=off  XmcBlockStatus=1  maskContainerNames=group1  block_type=delay  block_config=sysgen:Delay_config
  Delay1 : xbsIndex_r4/Delay  rst=off  en=off  latency=3  reg_retiming=off  XmcBlockStatus=1  maskContainerNames=group1  block_type=delay  block_config=sysgen:Delay_config
  Delay4 : xbsIndex_r4/Delay  rst=off  en=off  latency=27  reg_retiming=off  XmcBlockStatus=1  maskContainerNames=group1  block_type=delay  block_config=sysgen:Delay_config
  Gateway Out : xbsIndex_r4/Gateway Out  inherit_from_input=off  hdl_port=off  rows=1  columns=1  UseAsDAC=off  DACChannel='1'  interface=None  automatic_assignment=on  address_offset=hex2dec('00')  intf_name=''  intf_description=''  timing_constraint=None  locs_specified=off  LOCs={}  io_standard={}  XmcBlockStatus=1  maskContainerNames=group4  block_type=gatewayout  block_config=sysgen:gateway_out_config
  Gateway Out1 : xbsIndex_r4/Gateway Out  inherit_from_input=off  hdl_port=off  rows=1  columns=1  UseAsDAC=off  DACChannel='1'  interface=None  automatic_assignment=on  address_offset=hex2dec('00')  intf_name=''  intf_description=''  timing_constraint=None  locs_specified=off  LOCs={}  io_standard={}  XmcBlockStatus=1  maskContainerNames=group4  block_type=gatewayout  block_config=sysgen:gateway_out_config
  Real-Imag to Complex1 : RealImagToComplex
  Register : xbsIndex_r4/Register  init=0  rst=off  en=off  XmcBlockStatus=1  maskContainerNames=tabcontainer1  block_type=register  block_config=sysgen:Register_config
  Register1 : xbsIndex_r4/Register  init=0  rst=off  en=off  XmcBlockStatus=1  maskContainerNames=tabcontainer1  block_type=register  block_config=sysgen:Register_config
  Register2 : xbsIndex_r4/Register  init=0  rst=off  en=on  XmcBlockStatus=1  maskContainerNames=tabcontainer1  block_type=register  block_config=sysgen:Register_config
  Register3 : xbsIndex_r4/Register  init=0  rst=off  en=on  XmcBlockStatus=1  maskContainerNames=tabcontainer1  block_type=register  block_config=sysgen:Register_config
  Relational : xbsIndex_r4/Relational  mode=a=b  op_type=Bool  en=off  latency=0  XmcBlockStatus=1  maskContainerNames=tabcontainer1  block_type=relational  block_config=sysgen:Relational_config
  I_Out : Outport  VectorParamsAs1DForOutWhenUnconnected=off
  Q_Out : Outport  Port=2  VectorParamsAs1DForOutWhenUnconnected=off
  Coeff : Outport  Port=3  VectorParamsAs1DForOutWhenUnconnected=off
  wires:
  Q_In/1 -> Addressable Shift Register1/1
  I_In/1 -> Addressable Shift Register/1
  Addressable Shift Register1/1 -> Cmplx Mult w Ngtd BI/2(AI), Delay4/1
  Addressable Shift Register/1 -> Cmplx Mult w Ngtd BI/1(AR), Delay/1
  Register3/1 -> Q_Out/1
  Register2/1 -> I_Out/1
  Cmplx Mult1/1(PR) -> Register/1
  Cmplx Mult1/2(PI) -> Register1/1
  Err_Q/1 -> Cmplx Mult1/4(BI)
  Err_I/1 -> Cmplx Mult1/3(BR)
  Real-Imag to Complex1/1 -> Coeff/1
  Gateway Out1/1 -> Real-Imag to Complex1/2
  Gateway Out/1 -> Real-Imag to Complex1/1
  AddSub1/1 -> Coeff Buffer/1(In)
  AddSub2/1 -> Coeff Buffer1/1(In)
  Counter/1 -> Relational/1, Addressable Shift Register/2, Addressable Shift Register1/2
  Relational/1 -> Delay1/1
  Constant/1 -> Relational/2
  Coeff Buffer/1(Out) -> Gateway Out/1, Cmplx Mult w Ngtd BI/3(BR), AddSub1/2
  Coeff Buffer1/1(Out) -> AddSub2/2, Gateway Out1/1, Cmplx Mult w Ngtd BI/4(BI)
  Register/1 -> AddSub1/1
  Register1/1 -> AddSub2/1
  Accumulator1/1 -> Register3/1
  Cmplx Mult w Ngtd BI/2(PI) -> Accumulator1/1
  Cmplx Mult w Ngtd BI/1(PR) -> Accumulator/1
  Delay1/1 -> Accumulator/2, Accumulator1/2, Register2/2, Register3/2
  Accumulator/1 -> Register2/1
  Delay/1 -> Cmplx Mult1/1(AR)
  Delay4/1 -> Cmplx Mult1/2(AI)

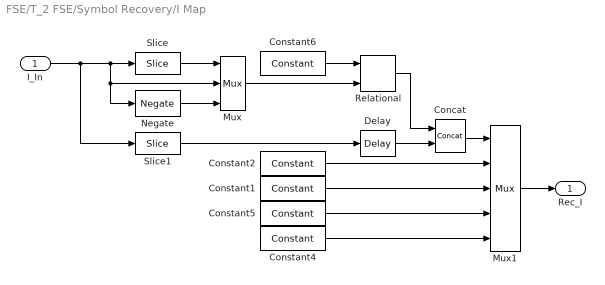
== system FSE/T_2 FSE/Symbol Recovery/I Map ==
  I_In : Inport
  Concat : xbsIndex_r4/Concat  num_inputs=2  XmcBlockStatus=1  maskContainerNames=group1  block_type=concat  block_config=sysgen:Concat_config
  Constant1 : xbsIndex_r4/Constant  const=-1/3  gui_display_data_type=Fixed-point  arith_type=Signed (2's comp)  n_bits=9  bin_pt=8  preci_type=Single  exp_width=8  frac_width=24  explicit_period=off  period=1  XmcBlockStatus=1  maskContainerNames=tabcontainer1  block_type=constant  block_config=sysgen:Constant_config
  Constant2 : xbsIndex_r4/Constant  const=1/3  gui_display_data_type=Fixed-point  arith_type=Signed (2's comp)  n_bits=9  bin_pt=8  preci_type=Single  exp_width=8  frac_width=24  explicit_period=off  period=1  XmcBlockStatus=1  maskContainerNames=tabcontainer1  block_type=constant  block_config=sysgen:Constant_config
  Constant4 : xbsIndex_r4/Constant  const=-1  gui_display_data_type=Fixed-point  arith_type=Signed (2's comp)  n_bits=2  bin_pt=0  preci_type=Single  exp_width=8  frac_width=24  explicit_period=off  period=1  XmcBlockStatus=1  maskContainerNames=tabcontainer1  block_type=constant  block_config=sysgen:Constant_config
  Constant5 : xbsIndex_r4/Constant  const=1  gui_display_data_type=Fixed-point  arith_type=Signed (2's comp)  n_bits=2  bin_pt=0  preci_type=Single  exp_width=8  frac_width=24  explicit_period=off  period=1  XmcBlockStatus=1  maskContainerNames=tabcontainer1  block_type=constant  block_config=sysgen:Constant_config
  Constant6 : xbsIndex_r4/Constant  const=2/3  gui_display_data_type=Fixed-point  arith_type=Unsigned  n_bits=8  bin_pt=8  preci_type=Single  exp_width=8  frac_width=24  explicit_period=off  period=1  XmcBlockStatus=1  maskContainerNames=tabcontainer1  block_type=constant  block_config=sysgen:Constant_config
  Delay : xbsIndex_r4/Delay  rst=off  en=off  latency=1  reg_retiming=off  XmcBlockStatus=1  maskContainerNames=group1  block_type=delay  block_config=sysgen:Delay_config
  Mux : xbsIndex_r4/Mux  inputs=2  en=off  latency=1  precision=Full  arith_type="Signed  (2's comp)"  n_bits=8  bin_pt=2  quantization=Truncate  overflow=Wrap  XmcBlockStatus=1  maskContainerNames=tabcontainer1  block_type=mux  block_config=sysgen:Mux_config
      settings: infoedit=[]
  Mux1 : xbsIndex_r4/Mux  inputs=4  en=off  latency=1  precision=User Defined  arith_type="Signed  (2's comp)"  n_bits=10  bin_pt=8  quantization=Truncate  overflow=Wrap  XmcBlockStatus=1  maskContainerNames=tabcontainer1  block_type=mux  block_config=sysgen:Mux_config
      settings: infoedit=[]
  Negate : xbsIndex_r4/Negate  precision=Full  arith_type=Unsigned  n_bits=18  bin_pt=10  quantization=Truncate  overflow=Wrap  en=off  latency=0  XmcBlockStatus=1  maskContainerNames=tabcontainer1  block_type=negate  block_config=sysgen:Negate_config
  Relational : xbsIndex_r4/Relational  mode=a<b  op_type=Bool  en=off  latency=0  XmcBlockStatus=1  maskContainerNames=tabcontainer1  block_type=relational  block_config=sysgen:Relational_config
  Slice : xbsIndex_r4/Slice  nbits=1  boolean_output=off  mode=Upper Bit Location + Width  bit1=0  base1=MSB of Input  bit0=0  base0=LSB of Input  XmcBlockStatus=1  maskContainerNames=group1  block_type=slice  block_config=sysgen:Slice_config
  Slice1 : xbsIndex_r4/Slice  nbits=1  boolean_output=off  mode=Upper Bit Location + Width  bit1=0  base1=MSB of Input  bit0=0  base0=LSB of Input  XmcBlockStatus=1  maskContainerNames=group1  block_type=slice  block_config=sysgen:Slice_config
  Rec_I : Outport  VectorParamsAs1DForOutWhenUnconnected=off
  wires:
  Mux1/1 -> Rec_I/1
  Concat/1 -> Mux1/1
  Constant5/1 -> Mux1/4
  Constant4/1 -> Mux1/5
  Constant1/1 -> Mux1/3
  Constant2/1 -> Mux1/2
  Slice/1 -> Mux/1
  I_In/1 -> Slice/1, Negate/1, Mux/2, Slice1/1
  Negate/1 -> Mux/3
  Mux/1 -> Relational/2
  Constant6/1 -> Relational/1
  Relational/1 -> Concat/1
  Slice1/1 -> Delay/1
  Delay/1 -> Concat/2
